simulink model "svpwm"  (R2021a)
settings: Solver=FixedStepDiscrete  StartTime=0.0  StopTime=10  FixedStep=1*10e-6  RelTol=1e-3
libraries: simulink x2
settings Model: Creator=Administrator  LastModifiedBy=Administrator

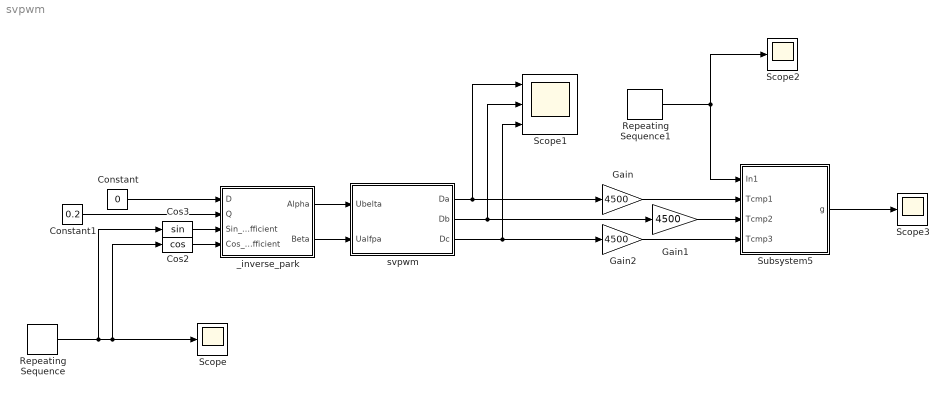
== system svpwm ==
  Constant : Constant  Value=0  OutDataTypeStr=single
  Constant1 : Constant  Value=0.2  OutDataTypeStr=single
  Cos2 : Trigonometry  Operator=cos
  Cos3 : Trigonometry
  Gain : Gain  Gain=4500
  Gain1 : Gain  Gain=4500
  Gain2 : Gain  Gain=4500
  Repeating Sequence : simulink/Sources/Repeating Sequence  rep_seq_t=[0 2]  rep_seq_y=[0 2*pi]
  Repeating Sequence1 : simulink/Sources/Repeating Sequence  rep_seq_t=[0 1/10000/2 1/10000]  rep_seq_y=[0 4500 0]
  Scope : Scope
  Scope1 : Scope  NumInputPorts=3
  Scope2 : Scope
  Scope3 : Scope
  Subsystem5 : Subsystem
  _inverse_park : Subsystem  TreatAsAtomicUnit=on
      settings: RTWSystemCode=Nonreusable function  RTWFcnNameOpts=Use subsystem name
      mask Display:
      | port_label('input',1,'D')
      | port_label('input',2,'Q')
      | port_label('input',3,'Sin')
      | port_label('input',4,'Cos')
      | port_label('output',1,'\alpha','texmode', 'on')
      | port_label('output',2,'\beta','texmode', 'on')
  svpwm : Subsystem
  wires:
  svpwm/1(Da) -> Scope1/1, Gain/1
  svpwm/2(Db) -> Gain1/1, Scope1/2
  svpwm/3(Dc) -> Gain2/1, Scope1/3
  _inverse_park/1(Alpha) -> svpwm/1(Ubelta)
  _inverse_park/2(Beta) -> svpwm/2(Ualfpa)
  Cos3/1 -> _inverse_park/3(Sin_Coefficient)
  Cos2/1 -> _inverse_park/4(Cos_Coefficient)
  Constant/1 -> _inverse_park/1(D)
  Constant1/1 -> _inverse_park/2(Q)
  Repeating Sequence/1 -> Scope/1, Cos2/1, Cos3/1
  Repeating Sequence1/1 -> Scope2/1, Subsystem5/1(In1)
  Gain/1 -> Subsystem5/2(Tcmp1)
  Gain1/1 -> Subsystem5/3(Tcmp2)
  Gain2/1 -> Subsystem5/4(Tcmp3)
  Subsystem5/1(g) -> Scope3/1

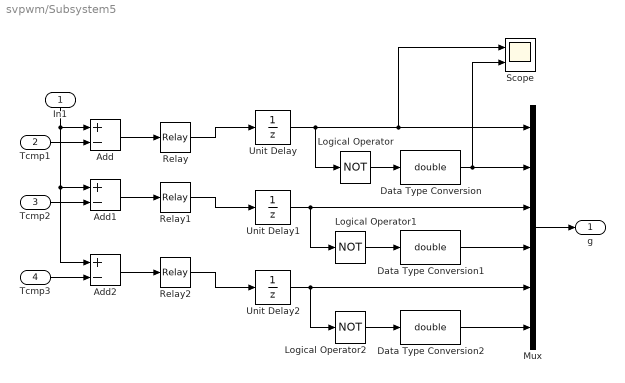
== system svpwm/Subsystem5 ==
  In1 : Inport
  Tcmp1 : Inport  Port=2
  Tcmp2 : Inport  Port=3
  Tcmp3 : Inport  Port=4
  Add : Sum  Inputs=+-
  Add1 : Sum  Inputs=+-
  Add2 : Sum  Inputs=+-
  Data Type Conversion : DataTypeConversion  OutDataTypeStr=double
  Data Type Conversion1 : DataTypeConversion  OutDataTypeStr=double
  Data Type Conversion2 : DataTypeConversion  OutDataTypeStr=double
  Logical Operator : Logic  Operator=NOT  AllPortsSameDT=off  OutDataTypeStr=boolean
  Logical Operator1 : Logic  Operator=NOT  AllPortsSameDT=off  OutDataTypeStr=boolean
  Logical Operator2 : Logic  Operator=NOT  AllPortsSameDT=off  OutDataTypeStr=boolean
  Mux : Mux  Inputs=6
  Relay : Relay  OffSwitchValue=-eps
  Relay1 : Relay  OffSwitchValue=-eps
  Relay2 : Relay  OffSwitchValue=-eps
  Scope : Scope  NumInputPorts=2
  Unit Delay : UnitDelay  SampleTime=-1  HasFrameUpgradeWarning=on
  Unit Delay1 : UnitDelay  SampleTime=-1  HasFrameUpgradeWarning=on
  Unit Delay2 : UnitDelay  SampleTime=-1  HasFrameUpgradeWarning=on
  g : Outport  VectorParamsAs1DForOutWhenUnconnected=off
  wires:
  Tcmp3/1 -> Add2/2
  Tcmp2/1 -> Add1/2
  Tcmp1/1 -> Add/2
  Relay2/1 -> Unit Delay2/1
  Relay1/1 -> Unit Delay1/1
  Relay/1 -> Unit Delay/1
  Unit Delay2/1 -> Mux/5, Logical Operator2/1
  Unit Delay1/1 -> Mux/3, Logical Operator1/1
  Unit Delay/1 -> Logical Operator/1, Scope/1, Mux/1
  Mux/1 -> g/1
  Data Type Conversion/1 -> Scope/2, Mux/2
  Data Type Conversion1/1 -> Mux/4
  Data Type Conversion2/1 -> Mux/6
  Logical Operator2/1 -> Data Type Conversion2/1
  Logical Operator1/1 -> Data Type Conversion1/1
  Logical Operator/1 -> Data Type Conversion/1
  Add1/1 -> Relay1/1
  Add2/1 -> Relay2/1
  Add/1 -> Relay/1
  In1/1 -> Add/1, Add2/1, Add1/1

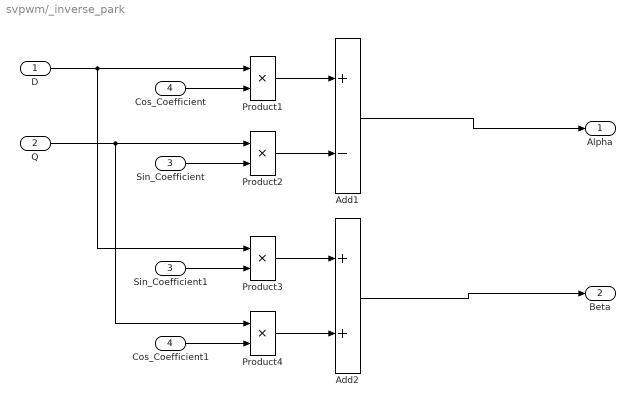
== system svpwm/_inverse_park ==
  D : Inport
  Q : Inport  Port=2
  Sin_Coefficient : Inport  Port=3
  Cos_Coefficient : Inport  Port=4
  Add1 : Sum  Inputs=+-  OutDataTypeStr=Inherit: Same as first input
  Add2 : Sum  OutDataTypeStr=Inherit: Same as first input
  Cos_Coefficient1 : InportShadow  Port=4
  Product{1..4} (4 alike) : Product  RndMeth=Simplest  OutDataTypeStr=Inherit: Same as first input
  Sin_Coefficient1 : InportShadow  Port=3
  Alpha : Outport  VectorParamsAs1DForOutWhenUnconnected=off
  Beta : Outport  Port=2  VectorParamsAs1DForOutWhenUnconnected=off
  wires:
  Product3/1 -> Add2/1
  Product4/1 -> Add2/2
  Product1/1 -> Add1/1
  Product2/1 -> Add1/2
  Cos_Coefficient1/1 -> Product4/2
  Sin_Coefficient/1 -> Product2/2
  D/1 -> Product3/1, Product1/1
  Q/1 -> Product2/1, Product4/1
  Sin_Coefficient1/1 -> Product3/2
  Cos_Coefficient/1 -> Product1/2
  Add1/1 -> Alpha/1
  Add2/1 -> Beta/1

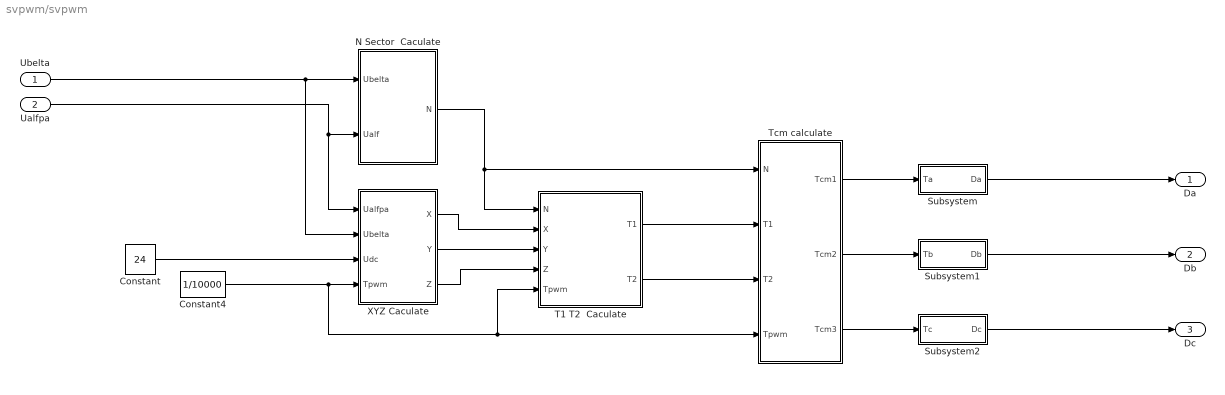
== system svpwm/svpwm ==
  Ubelta : Inport
  Ualfpa : Inport  Port=2
  Constant : Constant  Value=24  OutDataTypeStr=single
  Constant4 : Constant  Value=1/10000  OutDataTypeStr=single
  N Sector  Caculate : Subsystem  TreatAsAtomicUnit=on
  Subsystem : Subsystem
  Subsystem1 : Subsystem
  Subsystem2 : Subsystem
  T1 T2  Caculate : Subsystem  TreatAsAtomicUnit=on
  Tcm calculate : Subsystem  TreatAsAtomicUnit=on
  XYZ Caculate : Subsystem  TreatAsAtomicUnit=on
  Da : Outport
  Db : Outport  Port=2
  Dc : Outport  Port=3
  wires:
  XYZ Caculate/1(X) -> T1 T2  Caculate/2(X)
  Ubelta/1 -> N Sector  Caculate/1(Ubelta), XYZ Caculate/2(Ubelta)
  XYZ Caculate/2(Y) -> T1 T2  Caculate/3(Y)
  Constant4/1 -> XYZ Caculate/4(Tpwm), Tcm calculate/4(Tpwm), T1 T2  Caculate/5(Tpwm)
  Constant/1 -> XYZ Caculate/3(Udc)
  T1 T2  Caculate/1(T1) -> Tcm calculate/2(T1)
  Tcm calculate/1(Tcm1) -> Subsystem/1(Ta)
  Ualfpa/1 -> N Sector  Caculate/2(Ualf), XYZ Caculate/1(Ualfpa)
  XYZ Caculate/3(Z) -> T1 T2  Caculate/4(Z)
  N Sector  Caculate/1(N) -> T1 T2  Caculate/1(N), Tcm calculate/1(N)
  Tcm calculate/3(Tcm3) -> Subsystem2/1(Tc)
  T1 T2  Caculate/2(T2) -> Tcm calculate/3(T2)
  Tcm calculate/2(Tcm2) -> Subsystem1/1(Tb)
  Subsystem1/1(Db) -> Db/1
  Subsystem2/1(Dc) -> Dc/1
  Subsystem/1(Da) -> Da/1

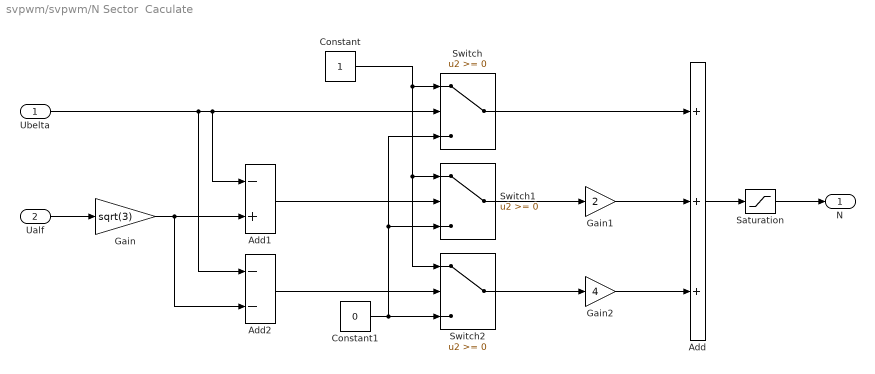
== system svpwm/svpwm/N Sector  Caculate ==
  Ubelta : Inport
  Ualf : Inport  Port=2
  Add : Sum  Inputs=+++
  Add1 : Sum  Inputs=-+  OutDataTypeStr=single
  Add2 : Sum  Inputs=--  OutDataTypeStr=single
  Constant : Constant  OutDataTypeStr=single
  Constant1 : Constant  Value=0  OutDataTypeStr=single
  Gain : Gain  Gain=sqrt(3)
  Gain1 : Gain  Gain=2
  Gain2 : Gain  Gain=4
  Saturation : Saturate  UpperLimit=6  LowerLimit=1
  Switch : Switch
  Switch1 : Switch
  Switch2 : Switch
  N : Outport
  wires:
  Saturation/1 -> N/1
  Add/1 -> Saturation/1
  Gain2/1 -> Add/3
  Switch2/1 -> Gain2/1
  Add2/1 -> Switch2/2
  Gain1/1 -> Add/2
  Switch1/1 -> Gain1/1
  Add1/1 -> Switch1/2
  Gain/1 -> Add2/2, Add1/2
  Ualf/1 -> Gain/1
  Switch/1 -> Add/1
  Constant1/1 -> Switch/3, Switch1/3, Switch2/3
  Constant/1 -> Switch/1, Switch1/1, Switch2/1
  Ubelta/1 -> Add2/1, Add1/1, Switch/2

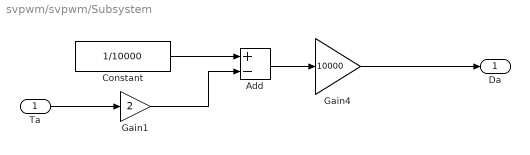
== system svpwm/svpwm/Subsystem ==
  Ta : Inport
  Add : Sum  Inputs=+-
  Constant : Constant  Value=1/10000  OutDataTypeStr=single
  Gain1 : Gain  Gain=2
  Gain4 : Gain  Gain=10000
  Da : Outport  OutDataTypeStr=single
  wires:
  Add/1 -> Gain4/1
  Gain1/1 -> Add/2
  Ta/1 -> Gain1/1
  Gain4/1 -> Da/1
  Constant/1 -> Add/1

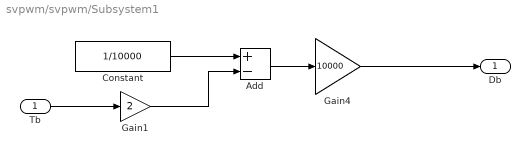
== system svpwm/svpwm/Subsystem1 ==
  Tb : Inport
  Add : Sum  Inputs=+-
  Constant : Constant  Value=1/10000  OutDataTypeStr=single
  Gain1 : Gain  Gain=2
  Gain4 : Gain  Gain=10000
  Db : Outport  OutDataTypeStr=single
  wires:
  Constant/1 -> Add/1
  Gain4/1 -> Db/1
  Tb/1 -> Gain1/1
  Gain1/1 -> Add/2
  Add/1 -> Gain4/1

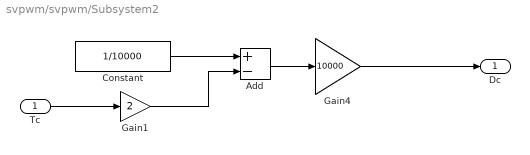
== system svpwm/svpwm/Subsystem2 ==
  Tc : Inport
  Add : Sum  Inputs=+-
  Constant : Constant  Value=1/10000  OutDataTypeStr=single
  Gain1 : Gain  Gain=2
  Gain4 : Gain  Gain=10000
  Dc : Outport  OutDataTypeStr=single
  wires:
  Add/1 -> Gain4/1
  Gain1/1 -> Add/2
  Tc/1 -> Gain1/1
  Gain4/1 -> Dc/1
  Constant/1 -> Add/1

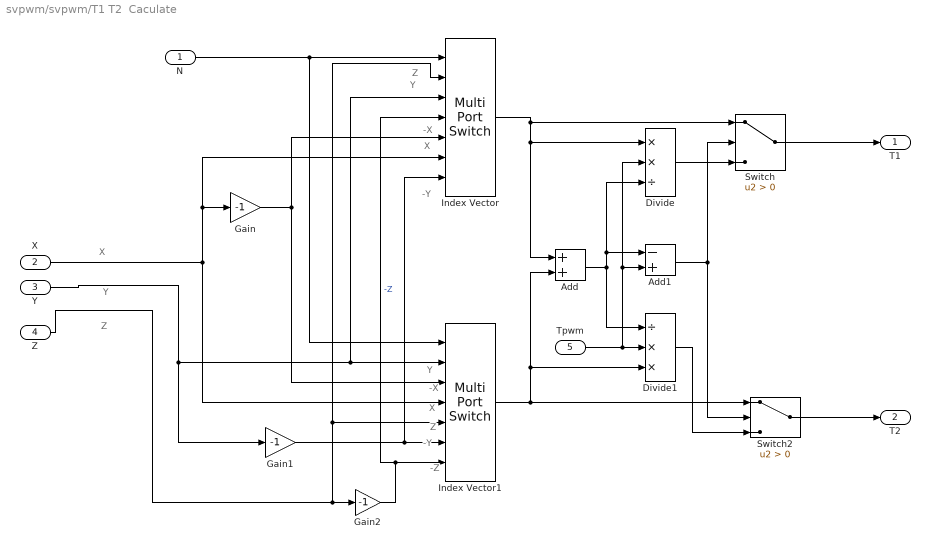
== system svpwm/svpwm/T1 T2  Caculate ==
  note: Z
  note: Y
  note: -X
  note: X
  note: -Y
  note: Y
  note: -X
  note: X
  note: Z
  note: -Y
  note: -Z
  note: X
  note: Y
  note: Z
  N : Inport
  X : Inport  Port=2
  Y : Inport  Port=3
  Z : Inport  Port=4
  Tpwm : Inport  Port=5
  Add : Sum
  Add1 : Sum  Inputs=-+
  Divide : Product  Inputs=**/
  Divide1 : Product  Inputs=/**
  Gain : Gain  Gain=-1
  Gain1 : Gain  Gain=-1
  Gain2 : Gain  Gain=-1
  Index Vector : MultiPortSwitch  Inputs=6
  Index Vector1 : MultiPortSwitch  Inputs=6
  Switch : Switch  Criteria=u2 > Threshold
  Switch2 : Switch  Criteria=u2 > Threshold
  T1 : Outport
  T2 : Outport  Port=2
  wires:
  Switch2/1 -> T2/1
  Divide1/1 -> Switch2/3
  Switch/1 -> T1/1
  Add1/1 -> Switch/2, Switch2/2
  Add/1 -> Divide1/1, Divide/3, Add1/1
  Tpwm/1 -> Divide1/2, Divide/2, Add1/2
  Divide/1 -> Switch/3
  Index Vector1/1 -> Switch2/1, Add/2, Divide1/3
  Index Vector/1 -> Switch/1, Divide/1, Add/1
  Gain1/1 -> Index Vector/7, Index Vector1/6
  Gain2/1 -> Index Vector/4, Index Vector1/7  "-Z"
  Gain/1 -> Index Vector/5, Index Vector1/3
  Y/1 -> Gain1/1, Index Vector/3, Index Vector1/2
  X/1 -> Index Vector1/4, Index Vector/6, Gain/1
  Z/1 -> Index Vector/2, Index Vector1/5, Gain2/1
  N/1 -> Index Vector1/1, Index Vector/1

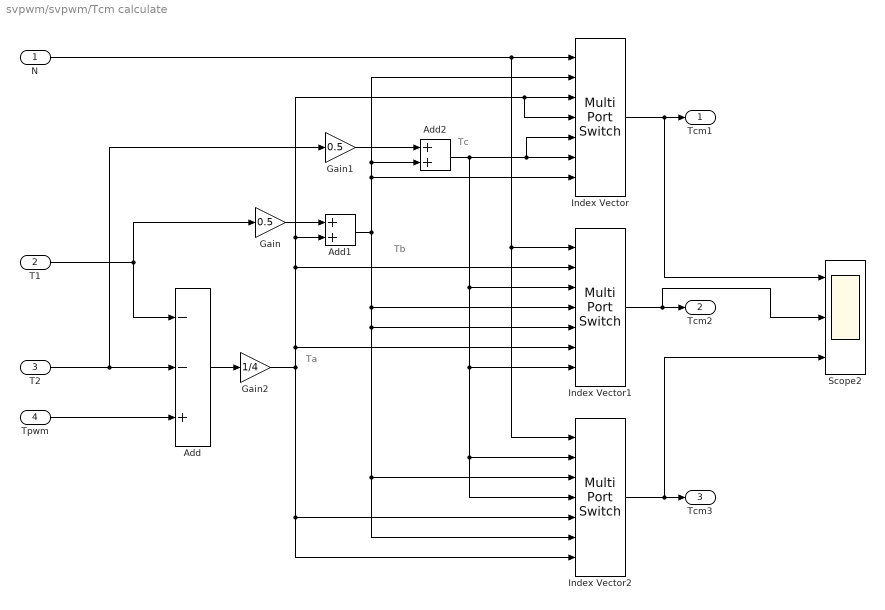
== system svpwm/svpwm/Tcm calculate ==
  note: Tc
  note: Tb
  note: Ta
  N : Inport
  T1 : Inport  Port=2
  T2 : Inport  Port=3
  Tpwm : Inport  Port=4
  Add : Sum  Inputs=--+
  Add1 : Sum
  Add2 : Sum
  Gain : Gain  Gain=0.5
  Gain1 : Gain  Gain=0.5
  Gain2 : Gain  Gain=1/4
  Index Vector : MultiPortSwitch  Inputs=6
  Index Vector1 : MultiPortSwitch  Inputs=6
  Index Vector2 : MultiPortSwitch  Inputs=6
  Scope2 : Scope  NumInputPorts=3
  Tcm1 : Outport
  Tcm2 : Outport  Port=2
  Tcm3 : Outport  Port=3
  wires:
  Index Vector2/1 -> Scope2/3, Tcm3/1
  N/1 -> Index Vector/1, Index Vector1/1, Index Vector2/1
  Add2/1 -> Index Vector/5, Index Vector/6, Index Vector1/3, Index Vector1/7, Index Vector2/2, Index Vector2/4
  Gain1/1 -> Add2/1
  Add1/1 -> Add2/2, Index Vector/2, Index Vector/7, Index Vector1/4, Index Vector1/5, Index Vector2/3, Index Vector2/6
  Gain2/1 -> Index Vector2/5, Index Vector2/7, Add1/2, Index Vector/3, Index Vector/4, Index Vector1/2, Index Vector1/6
  Gain/1 -> Add1/1
  Add/1 -> Gain2/1
  Tpwm/1 -> Add/3
  T2/1 -> Add/2, Gain1/1
  T1/1 -> Add/1, Gain/1
  Index Vector/1 -> Scope2/1, Tcm1/1
  Index Vector1/1 -> Scope2/2, Tcm2/1

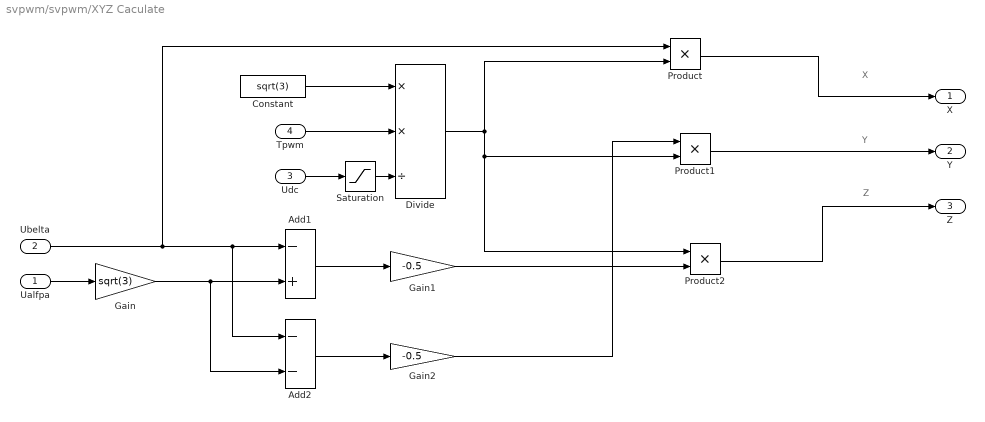
== system svpwm/svpwm/XYZ Caculate ==
  note: X
  note: Y
  note: Z
  Ualfpa : Inport
  Ubelta : Inport  Port=2
  Udc : Inport  Port=3
  Tpwm : Inport  Port=4
  Add1 : Sum  Inputs=-+
  Add2 : Sum  Inputs=--
  Constant : Constant  Value=sqrt(3)  OutDataTypeStr=single
  Divide : Product  Inputs=**/
  Gain : Gain  Gain=sqrt(3)
  Gain1 : Gain  Gain=-0.5
  Gain2 : Gain  Gain=-0.5
  Product : Product
  Product1 : Product
  Product2 : Product
  Saturation : Saturate  UpperLimit=1200  LowerLimit=0.0001
  X : Outport
  Y : Outport  Port=2
  Z : Outport  Port=3
  wires:
  Gain2/1 -> Product1/1
  Add2/1 -> Gain2/1
  Add1/1 -> Gain1/1
  Gain/1 -> Add2/2, Add1/2
  Ualfpa/1 -> Gain/1
  Ubelta/1 -> Add2/1, Add1/1, Product/1
  Gain1/1 -> Product2/2
  Product2/1 -> Z/1
  Divide/1 -> Product1/2, Product2/1, Product/2
  Product1/1 -> Y/1
  Product/1 -> X/1
  Udc/1 -> Saturation/1
  Tpwm/1 -> Divide/2
  Constant/1 -> Divide/1
  Saturation/1 -> Divide/3
